simulink model "ControlObsSemCanal"  (R2018a)
settings: Solver=VariableStepAuto  StartTime=0.0  StopTime=20.0  RelTol=1e-3
values from neighbouring files (symbols this model uses):
  C = GYzss.C    [ProjetoControl.m]    (also in ProjetoControlPI.m)
  F = acker(G, H, P)    [ProjetoControl.m]    (also in ProjetoControlPI.m = FKi(1:size(G,2)))
  G = GYzss.A    [ProjetoControl.m]    (also in ProjetoControlPI.m)
  H = GYzss.B    [ProjetoControl.m]    (also in ProjetoControlPI.m)
  Kc = 1/dcgain(SysCtl)    [ProjetoControl.m]    (also in ProjetoControlPI.m = 1/Y(end))
  L = L'    [ProjetoControl.m]    (also in ProjetoControlPI.m)
  Ts = 0.001*fd    (= 0.013)    [ProjetoControl.m]    (also in ProjetoControlPI.m)
settings Model: Creator=castr  LastModifiedBy=castr

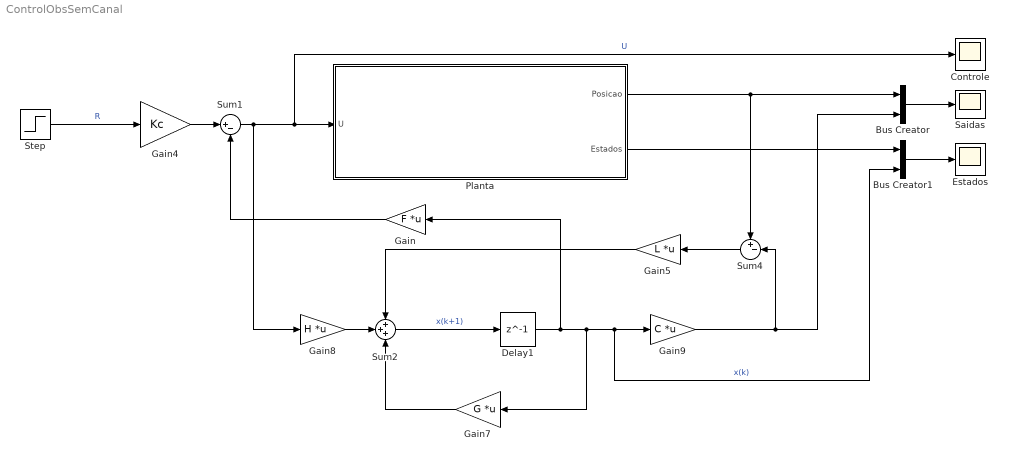
== system ControlObsSemCanal ==
  Bus Creator : BusCreator  Inputs=2
  Bus Creator1 : BusCreator  Inputs=2
  Controle : Scope
  Delay1 : Delay  DelayLength=1  SampleTime=Ts
  Estados : Scope
  Gain : Gain  Gain=F  Multiplication=Matrix(K*u)
  Gain4 : Gain  Gain=Kc
  Gain5 : Gain  Gain=L  Multiplication=Matrix(K*u)
  Gain7 : Gain  Gain=G  Multiplication=Matrix(K*u)
  Gain8 : Gain  Gain=H  Multiplication=Matrix(K*u)
  Gain9 : Gain  Gain=C  Multiplication=Matrix(K*u)
  Planta : Subsystem
  Saidas : Scope
  Step : Step  SampleTime=0
  Sum1 : Sum  Inputs=|+-
  Sum2 : Sum  Inputs=+++
  Sum4 : Sum  Inputs=+-|
  wires:
  Sum1/1 -> Gain8/1, Controle/1, Planta/1(U)  "U"
  Gain/1 -> Sum1/2
  Step/1 -> Gain4/1  "R"
  Bus Creator/1 -> Saidas/1
  Sum2/1 -> Delay1/1  "x(k+1)"
  Delay1/1 -> Gain/1, Gain9/1, Bus Creator1/2, Gain7/1  "x(k)"
  Gain4/1 -> Sum1/1
  Gain9/1 -> Sum4/2, Bus Creator/2
  Sum4/1 -> Gain5/1
  Gain7/1 -> Sum2/3
  Gain8/1 -> Sum2/2
  Gain5/1 -> Sum2/1
  Planta/1(Posicao) -> Sum4/1, Bus Creator/1
  Bus Creator1/1 -> Estados/1
  Planta/2(Estados) -> Bus Creator1/1

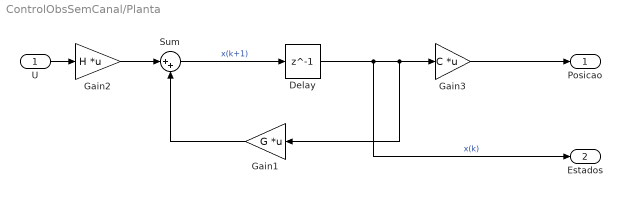
== system ControlObsSemCanal/Planta ==
  U : Inport
  Delay : Delay  DelayLength=1  InitialCondition=[0 0]  SampleTime=Ts
  Gain1 : Gain  Gain=G  Multiplication=Matrix(K*u)
  Gain2 : Gain  Gain=H  Multiplication=Matrix(K*u)
  Gain3 : Gain  Gain=C  Multiplication=Matrix(K*u)
  Sum : Sum  Inputs=|++
  Posicao : Outport
  Estados : Outport  Port=2
  wires:
  Gain1/1 -> Sum/2
  Gain2/1 -> Sum/1
  U/1 -> Gain2/1
  Sum/1 -> Delay/1  "x(k+1)"
  Delay/1 -> Estados/1, Gain1/1, Gain3/1  "x(k)"
  Gain3/1 -> Posicao/1
